simulink model "Cosim_Simulink"  (R2022b)
settings: Solver=FixedStepAuto  StartTime=0.0  StopTime=10  FixedStep=0.01  RelTol=1e-3
settings Model: Creator=charl  LastModifiedBy=charl

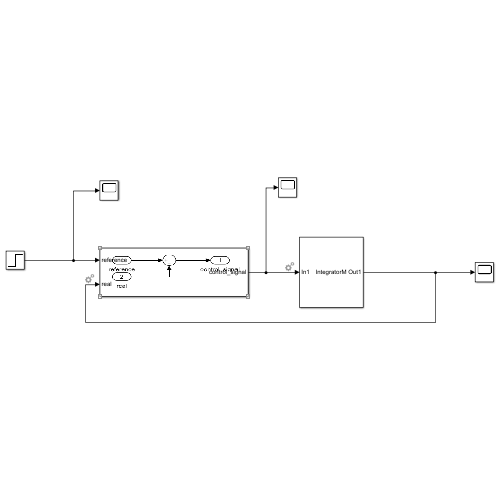
[thumbnail: Simulink's stored preview of the top-level diagram]
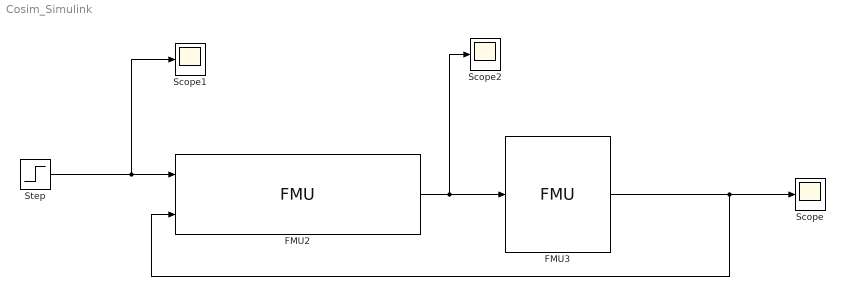
== system Cosim_Simulink ==
  FMU2 : FMU  FMUName=proportional_control.fmu  FMUMode=CoSimulation  FMUCreateBusObject=off
      mask Type: proportional_control [Co-Simulation, v2.0]
      mask Display:
      | if (exist([Simulink.fileGenControl('get','CacheFolder') '\slprj\_fmu\2ddf55bbe37cb6fbd3616df750eb4151\proportional_control\model.png'],'file'))
      |     image([Simulink.fileGenControl('get','CacheFolder') '\slprj\_fmu\2ddf55bbe37cb6fbd3616df750eb4151\proportional_control\model.png']);
      | else
      |     disp('proportional_control');
      | end
      | port_label('output',1,'control_signal');
      | port_label('input',1,'reference');
      | port_label('input',2,'real');
  FMU3 : FMU  FMUName=IntegratorM.fmu  FMUMode=CoSimulation  System=struct('k',1.0,'y_start',0.0)  mask(IntegratorM [Co-Simulation, v2.0]){}
      mask Display:
      | disp('IntegratorM');
      | port_label('output',1,'Out1');
      | port_label('input',1,'In1');
  Scope : Scope
  Scope1 : Scope
  Scope2 : Scope
  Step : Step  SampleTime=0
  wires:
  Step/1 -> Scope1/1, FMU2/1
  FMU2/1 -> Scope2/1, FMU3/1
  FMU3/1 -> Scope/1, FMU2/2
